simulink model "EKFfilter"  (R2016a)
settings: Solver=VariableStepAuto  StartTime=0.0  StopTime=100  RelTol=1e-3
libraries: simulink x2
settings Model: Creator=24535  LastModifiedBy=24535

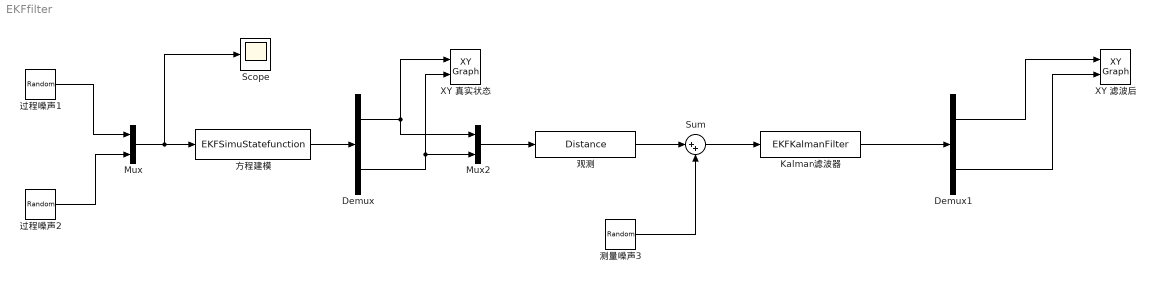
== system EKFfilter ==
  Demux : Demux  Outputs=2
  Demux1 : Demux  Outputs=2
  Kalman滤波器 : S-Function  FunctionName=EKFKalmanFilter  SFunctionDeploymentMode=off  EnableBusSupport=off
  Mux : Mux  Inputs=2
  Mux2 : Mux  Inputs=2
  Scope : Scope
  Sum : Sum  Inputs=|++
  XY 滤波后 : simulink/Sinks/XY Graph  xmin=0  xmax=50  ymin=-5  ymax=25  st=-1
  XY 真实状态 : simulink/Sinks/XY Graph  xmin=0  xmax=50  ymin=-5  ymax=25  st=-1
  方程建模 : S-Function  FunctionName=EKFSimuStatefunction  SFunctionDeploymentMode=off  EnableBusSupport=off
  测量噪声3 : RandomNumber  SampleTime=1
  观测 : S-Function  FunctionName=Distance  SFunctionDeploymentMode=off  EnableBusSupport=off
  过程噪声1 : RandomNumber  Variance=0.01  SampleTime=1
  过程噪声2 : RandomNumber  Variance=0.09  Seed=3  SampleTime=1
  wires:
  过程噪声1/1 -> Mux/1
  过程噪声2/1 -> Mux/2
  Mux/1 -> Scope/1, 方程建模/1
  方程建模/1 -> Demux/1
  Demux/1 -> Mux2/1, XY 真实状态/1
  Demux/2 -> Mux2/2, XY 真实状态/2
  Mux2/1 -> 观测/1
  观测/1 -> Sum/1
  Sum/1 -> Kalman滤波器/1
  测量噪声3/1 -> Sum/2
  Kalman滤波器/1 -> Demux1/1
  Demux1/1 -> XY 滤波后/1
  Demux1/2 -> XY 滤波后/2
